simulink model "Double_Link_Pendulum_Main"  (R2026a)
settings: Solver=FixedStepDiscrete  StopTime=12.49999999999999  FixedStep=0.1111111111111108
settings Model: Creator=H.Tam  LastModifiedBy=H.Tam

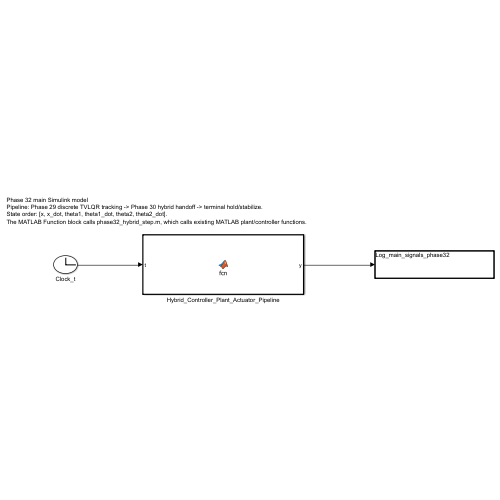
[thumbnail: Simulink's stored preview of the top-level diagram]
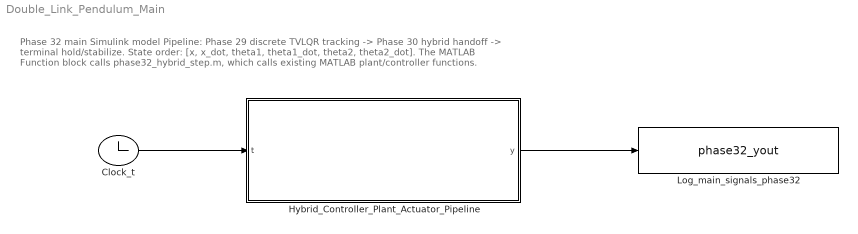
== system Double_Link_Pendulum_Main ==
  note: Phase 32 main Simulink model
      | Pipeline: Phase 29 discrete TVLQR tracking -> Phase 30 hybrid handoff -> terminal hold/stabilize.
      | State order: [x, x_dot, theta1, theta1_dot, theta2, theta2_dot].
      | The MATLAB Function block calls phase32_hybrid_step.m, which calls existing MATLAB plant/controller functions.
  Clock_t : Clock
  Hybrid_Controller_Plant_Actuator_Pipeline : MATLAB Function  TreatAsAtomicUnit=on
  Log_main_signals_phase32 : ToWorkspace  VariableName=phase32_yout  SaveFormat=Structure With Time  SampleTime=-1
  wires:
  Clock_t/1 -> Hybrid_Controller_Plant_Actuator_Pipeline/1(t)
  Hybrid_Controller_Plant_Actuator_Pipeline/1(y) -> Log_main_signals_phase32/1

== matlab function Double_Link_Pendulum_Main/Hybrid_Controller_Plant_Actuator_Pipeline ==
  data: t input; y output
function y = fcn(t)
%#codegen
coder.extrinsic('phase32_hybrid_step');
y = zeros(34,1);
tmp = phase32_hybrid_step(t,false);
y = tmp;
end
